simulink model "gtcs_mcb_v2"  (R2022a)
settings: Solver=VariableStepAuto  StartTime=0.0  StopTime=10  RelTol=1e-3
undefined symbols (not defined in the file or in its folder): gain
libraries: mcbplantlib x1, mcbcontrolslib x1, autolibpmsmexterior x1
settings Model: Creator=yusuf.ogut  LastModifiedBy=yusuf.ogut

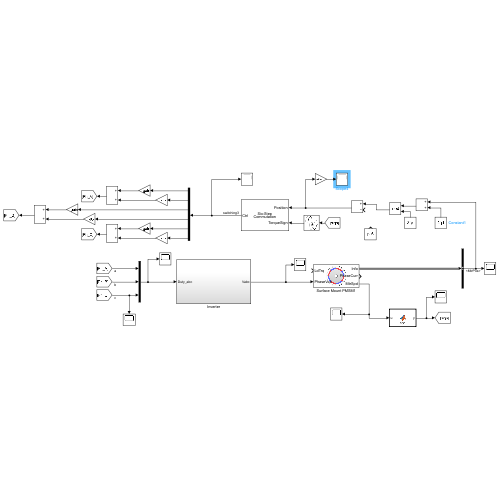
[thumbnail: Simulink's stored preview of the top-level diagram]
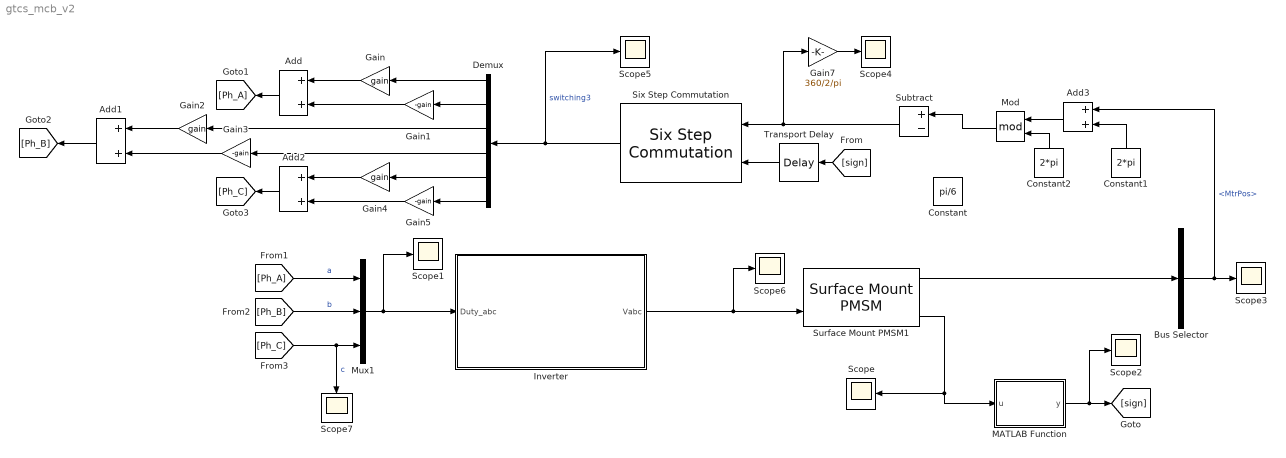
== system gtcs_mcb_v2 ==
  Add{,1..3} (4 alike) : Sum
  Bus Selector : BusSelector  OutputSignals=MtrPos
  Constant : Constant  Value=pi/6
  Constant1 : Constant  Value=2*pi
  Constant2 : Constant  Value=2*pi
  Demux : Demux  Outputs=6
  Gain : Gain  Gain=gain
  Gain1 : Gain  Gain=-gain
  Gain2 : Gain  Gain=gain
  Gain3 : Gain  Gain=-gain
  Gain4 : Gain  Gain=gain
  Gain5 : Gain  Gain=-gain
  Gain7 : Gain  Gain=360/2/pi
  Inverter : Subsystem
  MATLAB Function : MATLAB Function  TreatAsAtomicUnit=on
  Mod : Math  Operator=mod
  Mux1 : Mux  Inputs=3
  Scope{,1..7} (8 alike) : Scope
  Six Step Commutation : mcbcontrolslib/Six Step Commutation  InputType=Position  PositionUnit=Radians  CommutationMode=120 deg  SequencePos=[5,4,6,2,3,1]  EnableCustomSwitching=off  CommutationSeqPos=[0 0 1 0 0 1;0 1 1 0 0 0;0 1 0 0 1 0;0 0 0 1 1 0;1 0 0 1 0 0;1 0 0 0 0 1]  CommutationSeqNeg="[0  1  1  0  0  0;0  1  0  0  1  0;0  0  0  1  1  0;1  0  0  1  0  0;1  0  0  0  0  1;0  0  1  0  0  1;]"
      settings: SourceProductBaseCode=MT
  Subtract : Sum  Inputs=+-
  Surface Mount PMSM1 : autolibpmsmexterior/Surface Mount PMSM  port_config=Torque  sim_type=Continuous  Ts=0.001  P=1  Rs=0.015  Ldq_=1.7e-6  KConstText=Torque constant (Kt):  lambda_pm=0.2205  Ke=25  Kt=0.04  mechanical=[1, 0.01, 0]  idq0=[0 0]  theta_init=0  omega_init=0  KConst=0.04  lambda_pm_calc=0.026667  RefBlkName='autolibpmsmexterior/Surface Mount PMSM'  aMode=5  Ldq="[0.0017      0.0017]"
      settings: SourceProductBaseCode=PW,DR,MT,VE
  Transport Delay : TransportDelay  DelayTime=0.1
  wires:
  Inverter/1(Vabc) -> Surface Mount PMSM1/2, Scope6/1
  Surface Mount PMSM1/3 -> Scope/1, MATLAB Function/1(u)
  Surface Mount PMSM1/1 -> Bus Selector/1
  Bus Selector/1 -> Add3/1, Scope3/1  "<MtrPos>"
  MATLAB Function/1(y) -> Scope2/1, [sign]
  Six Step Commutation/1 -> Scope5/1, Demux/1  "switching3"
  Demux/1 -> Gain/1
  Demux/2 -> Gain1/1
  Gain/1 -> Add/1
  Gain1/1 -> Add/2
  Demux/4 -> Gain3/1
  Gain3/1 -> Add1/2
  Gain2/1 -> Add1/1
  Demux/3 -> Gain2/1
  Demux/6 -> Gain5/1
  Gain5/1 -> Add2/2
  Gain4/1 -> Add2/1
  Demux/5 -> Gain4/1
  Add/1 -> [Ph_A]
  Add1/1 -> [Ph_B]
  Add2/1 -> [Ph_C]
  Mux1/1 -> Inverter/1(Duty_abc), Scope1/1
  Subtract/1 -> Gain7/1, Six Step Commutation/1
  [Ph_B] -> Mux1/2  "b"
  [Ph_A] -> Mux1/1  "a"
  [Ph_C] -> Scope7/1, Mux1/3  "c"
  Gain7/1 -> Scope4/1
  [sign] -> Transport Delay/1
  Transport Delay/1 -> Six Step Commutation/2
  Constant1/1 -> Add3/2
  Add3/1 -> Mod/1
  Constant2/1 -> Mod/2
  Mod/1 -> Subtract/1

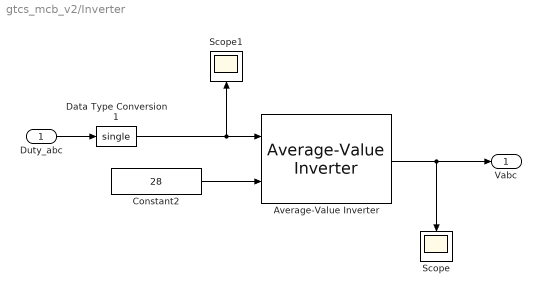
== system gtcs_mcb_v2/Inverter ==
  Duty_abc : Inport
  Average-Value Inverter : mcbplantlib/Average-Value Inverter
  Constant2 : Constant  Value=28  OutDataTypeStr=single  SampleTime=-1
  Data Type Conversion1 : DataTypeConversion  OutDataTypeStr=single  RndMeth=Simplest  SaturateOnIntegerOverflow=off
  Scope : Scope
  Scope1 : Scope
  Vabc : Outport  VectorParamsAs1DForOutWhenUnconnected=off
  wires:
  Constant2/1 -> Average-Value Inverter/2
  Duty_abc/1 -> Data Type Conversion1/1
  Data Type Conversion1/1 -> Scope1/1, Average-Value Inverter/1
  Average-Value Inverter/1 -> Scope/1, Vabc/1

== matlab function gtcs_mcb_v2/MATLAB Function ==
  data: u input; y output
function y = fcn(u)
    y = 1;
    if u<0
        y = -1;
    end
end
